simulink model "Practica1"  (R2022a)
settings: Solver=VariableStepAuto  StartTime=0.0  StopTime=60  RelTol=1e-3
settings Model: Creator=juanr  LastModifiedBy=juanr

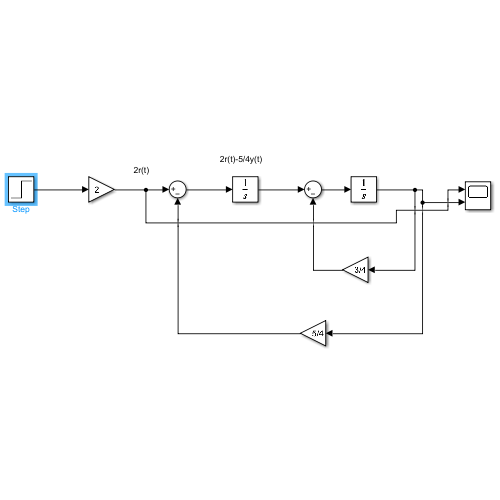
[thumbnail: Simulink's stored preview of the top-level diagram]
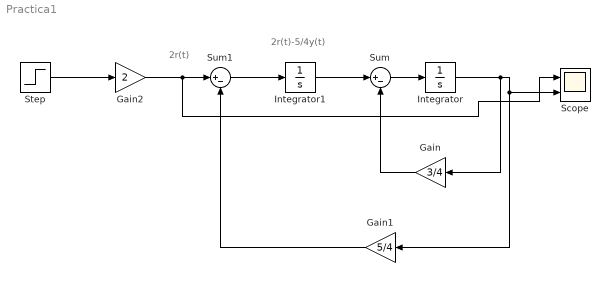
== system Practica1 ==
  note: 2r(t)-5/4y(t)
  note: 2r(t)
  Gain : Gain  Gain=3/4
  Gain1 : Gain  Gain=5/4
  Gain2 : Gain  Gain=2
  Integrator : Integrator
  Integrator1 : Integrator
  Scope : Scope  NumInputPorts=2
  Step : Step  SampleTime=0
  Sum : Sum  Inputs=|+-
  Sum1 : Sum  Inputs=|+-
  wires:
  Sum/1 -> Integrator/1
  Gain/1 -> Sum/2
  Integrator1/1 -> Sum/1
  Sum1/1 -> Integrator1/1
  Gain1/1 -> Sum1/2
  Step/1 -> Gain2/1
  Gain2/1 -> Scope/1, Sum1/1
  Integrator/1 -> Scope/2, Gain1/1, Gain/1
